simulink model "torqueBalancing2015a"  (Simulink 8.5)
settings: Solver=FixedStepDiscrete  StartTime=0.0  StopTime="CONFIG.SIMULATION_TIME "  FixedStep=CONFIG.Ts  RelTol=1e-3
InitFcn:
  | cd(fileparts(which(bdroot)));
  | initTorqueBalancing;
values from neighbouring files (symbols this model uses):
  WBT_modelName = 'matlabTorqueBalancing'    [initTorqueBalancing.m]
undefined symbols (not defined in the file or in its folder): bVectorConstraintsFeet, bVectorConstraintsLegs, CONFIG, ConstraintsMatrixFeet, ConstraintsMatrixLegs, DiscIntNeverNeededParam, gain, references, reg, ROBOT_DOF, ROBOT_DOF_FOR_SIMULINK, sat, SM, sm, WBT_robotName
libraries: WBToolboxLibrary x179, simulink x13
(part 3 of 4)

== system torqueBalancing2015a/DesValues/State Machine StandUp/w_H_root_link2 ==
  qj : Inport
  inertial : Inport  Port=2
  "CoM6D ->  CoMXYZ1" : Selector  NumberOfDimensions=2  InputPortWidth=7  IndexOptions=Index vector (dialog),Index vector (dialog)  Indices=[1 2 3],[1 2 3]  OutputSizes=1,1
  Constant2 : Constant  Value=eye(4)
  Constant5 : Constant  Value=eye(4)
  Constant6 : Constant  Value=eye(4)
  Inv\* : Product  Inputs=/*  Multiplication=Matrix(*)
  Inv\*1 : Product  Inputs=/*  Multiplication=Matrix(*)
  Inv\*2 : Product  Inputs=/  Multiplication=Matrix(*)
  Product : Product  Multiplication=Matrix(*)
  Selector : Selector  InputPortWidth=12  IndexOptions=Index vector (dialog)  Indices=[4 5 6 ]  OutputSizes=1
  Subsystem : Subsystem
  Switch6 : Switch  Criteria=u2 > Threshold
  USE_IMU4EST_BASE : Constant  Value=CONFIG.USE_IMU4EST_BASE
  fromImuToHomogeousTransformFCN : MATLAB Function  TreatAsAtomicUnit=on
      settings: PermitHierarchicalResolution=ParametersOnly
  holder 1 : WBToolboxLibrary/Utilities/holder 
  holder 2 : WBToolboxLibrary/Utilities/holder 
  imu : WBToolboxLibrary/wholeBodyModel/Kinematics/Forward Kinematics  frameName='imu_frame'  robotName=WBT_robotName  localName=WBT_modelName  wbiFile=WBT_wbiFilename  wbiList=WBT_wbiList
  l_sole_acc : Scope
      settings: TimeRange=60  ShowLegends=on  MaxDataPoints=5000  SaveToWorkspace=off  YMin=-4.47309  YMax=14.2668  SampleTime=-1
  link : WBToolboxLibrary/wholeBodyModel/Kinematics/Forward Kinematics  frameName=link_name  robotName=WBT_robotName  localName=WBT_modelName  wbiFile=WBT_wbiFilename  wbiList=WBT_wbiList
  root_link : WBToolboxLibrary/wholeBodyModel/Kinematics/Forward Kinematics  frameName='root_link'  robotName=WBT_robotName  localName=WBT_modelName  wbiFile=WBT_wbiFilename  wbiList=WBT_wbiList
  w_H_root : Outport
  wires:
  Constant5/1 -> imu/1
  Inv\*/1 -> holder 1/1, fromImuToHomogeousTransformFCN/1(imu_H_link), Inv\*2/1  "imu_H_link"
  imu/1 -> Inv\*/1
  Constant6/1 -> link/1
  Inv\*1/1 -> Switch6/3, fromImuToHomogeousTransformFCN/3(link_H_root)  "link_H_root"
  link/1 -> Inv\*1/1, Inv\*/2
  inertial/1 -> Selector/1, holder 2/1, fromImuToHomogeousTransformFCN/5(inertial)
  Switch6/1 -> w_H_root/1
  USE_IMU4EST_BASE/1 -> Switch6/2
  fromImuToHomogeousTransformFCN/1(w_H_root) -> Switch6/1
  Constant2/1 -> root_link/1
  qj/1 -> root_link/2, link/2, imu/2
  root_link/1 -> Inv\*1/2
  holder 1/1 -> fromImuToHomogeousTransformFCN/2(imu_H_link_0)
  holder 2/1 -> fromImuToHomogeousTransformFCN/4(inertial_0)
  Inv\*2/1 -> "CoM6D ->  CoMXYZ1"/1
  "CoM6D ->  CoMXYZ1"/1 -> Product/1  "l_sole_R_imu"
  Selector/1 -> Product/2  "imu_acce"
  Product/1 -> l_sole_acc/1
  Subsystem/1(Neck Position) -> fromImuToHomogeousTransformFCN/6(neck)

== system torqueBalancing2015a/DesValues/State Machine StandUp/xCom2 ==
  qj : Inport
  w_H_b : Inport  Port=2
  "CoM6D ->  CoMXYZ2" : Selector  NumberOfDimensions=2  InputPortWidth=7  IndexOptions=Index vector (dialog),Index vector (dialog)  Indices=[1 2 3],[4]  OutputSizes=1,1
  com : WBToolboxLibrary/wholeBodyModel/Kinematics/Forward Kinematics  frameName='com'  robotName=WBT_robotName  localName=WBT_modelName  wbiFile=WBT_wbiFilename  wbiList=WBT_wbiList
  xCom : Outport
  wires:
  qj/1 -> com/2
  "CoM6D ->  CoMXYZ2"/1 -> xCom/1
  com/1 -> "CoM6D ->  CoMXYZ2"/1
  w_H_b/1 -> com/1

== system torqueBalancing2015a/DesValues/State Machine Walking/Visualise extrnal wrenches   ==
  wL_WBDT : Inport
  wR_WBDT : Inport  Port=2
  Enable : EnablePort
  left foot ext wrench : Scope
      settings: TimeRange=auto  LimitDataPoints=on  MaxDataPoints=5000  SaveToWorkspace=off  YMin=-10  YMax=10  SampleTime=-1  DataFormat=Array
  right foot ext wrench : Scope
      settings: TimeRange=42.68  ShowLegends=on  MaxDataPoints=5000  SaveToWorkspace=off  SaveName=ScopeData2  YMin=-499.56546  YMax=285.33819  SampleTime=-1  DataFormat=Array
  wires:
  wR_WBDT/1 -> right foot ext wrench/1  "wR_WBDT"
  wL_WBDT/1 -> left foot ext wrench/1  "wL_WBDT"

== system torqueBalancing2015a/DesValues/State Machine Walking/nu ==
  qj : Inport
  w_H_b : Inport  Port=2
  "constraints " : Inport  Port=3
  Get Estimate : WBToolboxLibrary/wholeBodyStates/Get Estimate  estimateType=Joints Velocity  robotName=WBT_robotName  localName=WBT_modelName  wbiFile=WBT_wbiFilename  wbiList=WBT_wbiList
  Jacobian l_sole : WBToolboxLibrary/wholeBodyModel/Jacobians/Jacobian  frameName='l_sole'  robotName=WBT_robotName  localName=WBT_modelName  wbiFile=WBT_wbiFilename  wbiList=WBT_wbiList
  Jacobian r_sole : WBToolboxLibrary/wholeBodyModel/Jacobians/Jacobian  frameName='r_sole'  robotName=WBT_robotName  localName=WBT_modelName  wbiFile=WBT_wbiFilename  wbiList=WBT_wbiList
  MATLAB Function : MATLAB Function  TreatAsAtomicUnit=on
      settings: PermitHierarchicalResolution=ParametersOnly
  Mux : Mux  Inputs=2
  vb + Dqj : Outport
  wires:
  Get Estimate/1 -> MATLAB Function/4(qD), Mux/2
  Mux/1 -> vb + Dqj/1
  Jacobian r_sole/1 -> MATLAB Function/2(JcRightFoot)
  "constraints "/1 -> MATLAB Function/3(activeFeetConstraints)
  MATLAB Function/1(y) -> Mux/1
  Jacobian l_sole/1 -> MATLAB Function/1(JcLeftFoot)
  qj/1 -> Jacobian l_sole/2, Jacobian r_sole/2
  w_H_b/1 -> Jacobian r_sole/1, Jacobian l_sole/1

== system torqueBalancing2015a/DesValues/State Machine Walking/w_H_root_link1 ==
  qj : Inport
  inertial : Inport  Port=2
  "CoM6D ->  CoMXYZ1" : Selector  NumberOfDimensions=2  InputPortWidth=7  IndexOptions=Index vector (dialog),Index vector (dialog)  Indices=[1 2 3],[1 2 3]  OutputSizes=1,1
  Constant2 : Constant  Value=eye(4)
  Constant5 : Constant  Value=eye(4)
  Constant6 : Constant  Value=eye(4)
  Inv\* : Product  Inputs=/*  Multiplication=Matrix(*)
  Inv\*1 : Product  Inputs=/*  Multiplication=Matrix(*)
  Inv\*2 : Product  Inputs=/  Multiplication=Matrix(*)
  Product : Product  Multiplication=Matrix(*)
  Selector : Selector  InputPortWidth=12  IndexOptions=Index vector (dialog)  Indices=[4 5 6 ]  OutputSizes=1
  Subsystem : Subsystem
  Switch6 : Switch  Criteria=u2 > Threshold
  USE_IMU4EST_BASE : Constant  Value=CONFIG.USE_IMU4EST_BASE
  fromImuToHomogeousTransformFCN : MATLAB Function  TreatAsAtomicUnit=on
      settings: PermitHierarchicalResolution=ParametersOnly
  holder 1 : WBToolboxLibrary/Utilities/holder 
  holder 2 : WBToolboxLibrary/Utilities/holder 
  imu : WBToolboxLibrary/wholeBodyModel/Kinematics/Forward Kinematics  frameName='imu_frame'  robotName=WBT_robotName  localName=WBT_modelName  wbiFile=WBT_wbiFilename  wbiList=WBT_wbiList
  l_sole_acc : Scope
      settings: TimeRange=60  ShowLegends=on  MaxDataPoints=5000  SaveToWorkspace=off  YMin=-4.47309  YMax=14.2668  SampleTime=-1
  link : WBToolboxLibrary/wholeBodyModel/Kinematics/Forward Kinematics  frameName=link_name  robotName=WBT_robotName  localName=WBT_modelName  wbiFile=WBT_wbiFilename  wbiList=WBT_wbiList
  root_link : WBToolboxLibrary/wholeBodyModel/Kinematics/Forward Kinematics  frameName='root_link'  robotName=WBT_robotName  localName=WBT_modelName  wbiFile=WBT_wbiFilename  wbiList=WBT_wbiList
  w_H_root : Outport
  wires:
  Constant5/1 -> imu/1
  Inv\*/1 -> holder 1/1, fromImuToHomogeousTransformFCN/1(imu_H_link), Inv\*2/1  "imu_H_link"
  imu/1 -> Inv\*/1
  Constant6/1 -> link/1
  Inv\*1/1 -> Switch6/3, fromImuToHomogeousTransformFCN/3(link_H_root)  "link_H_root"
  link/1 -> Inv\*1/1, Inv\*/2
  inertial/1 -> Selector/1, holder 2/1, fromImuToHomogeousTransformFCN/5(inertial)
  Switch6/1 -> w_H_root/1
  USE_IMU4EST_BASE/1 -> Switch6/2
  fromImuToHomogeousTransformFCN/1(w_H_root) -> Switch6/1
  Constant2/1 -> root_link/1
  qj/1 -> root_link/2, link/2, imu/2
  root_link/1 -> Inv\*1/2
  holder 1/1 -> fromImuToHomogeousTransformFCN/2(imu_H_link_0)
  holder 2/1 -> fromImuToHomogeousTransformFCN/4(inertial_0)
  Inv\*2/1 -> "CoM6D ->  CoMXYZ1"/1
  "CoM6D ->  CoMXYZ1"/1 -> Product/1  "l_sole_R_imu"
  Selector/1 -> Product/2  "imu_acce"
  Product/1 -> l_sole_acc/1
  Subsystem/1(Neck Position) -> fromImuToHomogeousTransformFCN/6(neck)

== system torqueBalancing2015a/DesValues/State Machine Walking/w_H_root_link2 ==
  qj : Inport
  inertial : Inport  Port=2
  "CoM6D ->  CoMXYZ1" : Selector  NumberOfDimensions=2  InputPortWidth=7  IndexOptions=Index vector (dialog),Index vector (dialog)  Indices=[1 2 3],[1 2 3]  OutputSizes=1,1
  Constant2 : Constant  Value=eye(4)
  Constant5 : Constant  Value=eye(4)
  Constant6 : Constant  Value=eye(4)
  Inv\* : Product  Inputs=/*  Multiplication=Matrix(*)
  Inv\*1 : Product  Inputs=/*  Multiplication=Matrix(*)
  Inv\*2 : Product  Inputs=/  Multiplication=Matrix(*)
  Product : Product  Multiplication=Matrix(*)
  Selector : Selector  InputPortWidth=12  IndexOptions=Index vector (dialog)  Indices=[4 5 6 ]  OutputSizes=1
  Subsystem : Subsystem
  Switch6 : Switch  Criteria=u2 > Threshold
  USE_IMU4EST_BASE : Constant  Value=CONFIG.USE_IMU4EST_BASE
  fromImuToHomogeousTransformFCN : MATLAB Function  TreatAsAtomicUnit=on
      settings: PermitHierarchicalResolution=ParametersOnly
  holder 1 : WBToolboxLibrary/Utilities/holder 
  holder 2 : WBToolboxLibrary/Utilities/holder 
  imu : WBToolboxLibrary/wholeBodyModel/Kinematics/Forward Kinematics  frameName='imu_frame'  robotName=WBT_robotName  localName=WBT_modelName  wbiFile=WBT_wbiFilename  wbiList=WBT_wbiList
  l_sole_acc : Scope
      settings: TimeRange=60  ShowLegends=on  MaxDataPoints=5000  SaveToWorkspace=off  YMin=-4.47309  YMax=14.2668  SampleTime=-1
  link : WBToolboxLibrary/wholeBodyModel/Kinematics/Forward Kinematics  frameName=link_name  robotName=WBT_robotName  localName=WBT_modelName  wbiFile=WBT_wbiFilename  wbiList=WBT_wbiList
  root_link : WBToolboxLibrary/wholeBodyModel/Kinematics/Forward Kinematics  frameName='root_link'  robotName=WBT_robotName  localName=WBT_modelName  wbiFile=WBT_wbiFilename  wbiList=WBT_wbiList
  w_H_root : Outport
  wires:
  Constant5/1 -> imu/1
  Inv\*/1 -> holder 1/1, fromImuToHomogeousTransformFCN/1(imu_H_link), Inv\*2/1  "imu_H_link"
  imu/1 -> Inv\*/1
  Constant6/1 -> link/1
  Inv\*1/1 -> Switch6/3, fromImuToHomogeousTransformFCN/3(link_H_root)  "link_H_root"
  link/1 -> Inv\*1/1, Inv\*/2
  inertial/1 -> Selector/1, holder 2/1, fromImuToHomogeousTransformFCN/5(inertial)
  Switch6/1 -> w_H_root/1
  USE_IMU4EST_BASE/1 -> Switch6/2
  fromImuToHomogeousTransformFCN/1(w_H_root) -> Switch6/1
  Constant2/1 -> root_link/1
  qj/1 -> root_link/2, link/2, imu/2
  root_link/1 -> Inv\*1/2
  holder 1/1 -> fromImuToHomogeousTransformFCN/2(imu_H_link_0)
  holder 2/1 -> fromImuToHomogeousTransformFCN/4(inertial_0)
  Inv\*2/1 -> "CoM6D ->  CoMXYZ1"/1
  "CoM6D ->  CoMXYZ1"/1 -> Product/1  "l_sole_R_imu"
  Selector/1 -> Product/2  "imu_acce"
  Product/1 -> l_sole_acc/1
  Subsystem/1(Neck Position) -> fromImuToHomogeousTransformFCN/6(neck)

== system torqueBalancing2015a/DesValues/State Machine Walking/xCom ==
  qj : Inport
  w_H_b : Inport  Port=2
  "CoM6D ->  CoMXYZ2" : Selector  NumberOfDimensions=2  InputPortWidth=7  IndexOptions=Index vector (dialog),Index vector (dialog)  Indices=[1 2 3],[4]  OutputSizes=1,1
  com : WBToolboxLibrary/wholeBodyModel/Kinematics/Forward Kinematics  frameName='com'  robotName=WBT_robotName  localName=WBT_modelName  wbiFile=WBT_wbiFilename  wbiList=WBT_wbiList
  xCom : Outport
  wires:
  qj/1 -> com/2
  "CoM6D ->  CoMXYZ2"/1 -> xCom/1
  com/1 -> "CoM6D ->  CoMXYZ2"/1
  w_H_b/1 -> com/1

== system torqueBalancing2015a/DesValues/State Machine Walking/xCom1 ==
  qj : Inport
  w_H_b : Inport  Port=2
  "CoM6D ->  CoMXYZ2" : Selector  NumberOfDimensions=2  InputPortWidth=7  IndexOptions=Index vector (dialog),Index vector (dialog)  Indices=[1 2 3],[4]  OutputSizes=1,1
  com : WBToolboxLibrary/wholeBodyModel/Kinematics/Forward Kinematics  frameName='com'  robotName=WBT_robotName  localName=WBT_modelName  wbiFile=WBT_wbiFilename  wbiList=WBT_wbiList
  xCom : Outport
  wires:
  qj/1 -> com/2
  "CoM6D ->  CoMXYZ2"/1 -> xCom/1
  com/1 -> "CoM6D ->  CoMXYZ2"/1
  w_H_b/1 -> com/1

== system torqueBalancing2015a/controller_QP/QP/Visualize eventual QP failures ==
  exitFlagQP : Inport
  state : Inport  Port=2
  Enable : EnablePort
  "QP status (0: no failure, 1: not using)" : Scope  NumInputPorts=2
      settings: TimeRange=auto  ShowLegends=on  MaxDataPoints=5000  SaveName=QPStatus  YMin=-2.25~0.625  YMax=0.25~4.375  SampleTime=-1
  wires:
  exitFlagQP/1 -> "QP status (0: no failure, 1: not using)"/1  "exitFlagQP"
  state/1 -> "QP status (0: no failure, 1: not using)"/2

== system torqueBalancing2015a/controller_QP/integralOf Hw1/w_H_root_link1 ==
  qj : Inport
  inertial : Inport  Port=2
  "CoM6D ->  CoMXYZ1" : Selector  NumberOfDimensions=2  InputPortWidth=7  IndexOptions=Index vector (dialog),Index vector (dialog)  Indices=[1 2 3],[1 2 3]  OutputSizes=1,1
  Constant2 : Constant  Value=eye(4)
  Constant5 : Constant  Value=eye(4)
  Constant6 : Constant  Value=eye(4)
  Inv\* : Product  Inputs=/*  Multiplication=Matrix(*)
  Inv\*1 : Product  Inputs=/*  Multiplication=Matrix(*)
  Inv\*2 : Product  Inputs=/  Multiplication=Matrix(*)
  Product : Product  Multiplication=Matrix(*)
  Selector : Selector  InputPortWidth=12  IndexOptions=Index vector (dialog)  Indices=[4 5 6 ]  OutputSizes=1
  Subsystem : Subsystem
  Switch6 : Switch  Criteria=u2 > Threshold
  USE_IMU4EST_BASE : Constant  Value=CONFIG.USE_IMU4EST_BASE
  fromImuToHomogeousTransformFCN : MATLAB Function  TreatAsAtomicUnit=on
      settings: PermitHierarchicalResolution=ParametersOnly
  holder 1 : WBToolboxLibrary/Utilities/holder 
  holder 2 : WBToolboxLibrary/Utilities/holder 
  imu : WBToolboxLibrary/wholeBodyModel/Kinematics/Forward Kinematics  frameName='imu_frame'  robotName=WBT_robotName  localName=WBT_modelName  wbiFile=WBT_wbiFilename  wbiList=WBT_wbiList
  l_sole_acc : Scope
      settings: TimeRange=60  ShowLegends=on  MaxDataPoints=5000  SaveToWorkspace=off  YMin=-4.47309  YMax=14.2668  SampleTime=-1
  link : WBToolboxLibrary/wholeBodyModel/Kinematics/Forward Kinematics  frameName=link_name  robotName=WBT_robotName  localName=WBT_modelName  wbiFile=WBT_wbiFilename  wbiList=WBT_wbiList
  root_link : WBToolboxLibrary/wholeBodyModel/Kinematics/Forward Kinematics  frameName='root_link'  robotName=WBT_robotName  localName=WBT_modelName  wbiFile=WBT_wbiFilename  wbiList=WBT_wbiList
  w_H_root : Outport
  wires:
  Constant5/1 -> imu/1
  Inv\*/1 -> holder 1/1, fromImuToHomogeousTransformFCN/1(imu_H_link), Inv\*2/1  "imu_H_link"
  imu/1 -> Inv\*/1
  Constant6/1 -> link/1
  Inv\*1/1 -> Switch6/3, fromImuToHomogeousTransformFCN/3(link_H_root)  "link_H_root"
  link/1 -> Inv\*1/1, Inv\*/2
  inertial/1 -> Selector/1, holder 2/1, fromImuToHomogeousTransformFCN/5(inertial)
  Switch6/1 -> w_H_root/1
  USE_IMU4EST_BASE/1 -> Switch6/2
  fromImuToHomogeousTransformFCN/1(w_H_root) -> Switch6/1
  Constant2/1 -> root_link/1
  qj/1 -> root_link/2, link/2, imu/2
  root_link/1 -> Inv\*1/2
  holder 1/1 -> fromImuToHomogeousTransformFCN/2(imu_H_link_0)
  holder 2/1 -> fromImuToHomogeousTransformFCN/4(inertial_0)
  Inv\*2/1 -> "CoM6D ->  CoMXYZ1"/1
  "CoM6D ->  CoMXYZ1"/1 -> Product/1  "l_sole_R_imu"
  Selector/1 -> Product/2  "imu_acce"
  Product/1 -> l_sole_acc/1
  Subsystem/1(Neck Position) -> fromImuToHomogeousTransformFCN/6(neck)

== system torqueBalancing2015a/controller_QP/integralOf Hw1/w_H_root_link2 ==
  qj : Inport
  inertial : Inport  Port=2
  "CoM6D ->  CoMXYZ1" : Selector  NumberOfDimensions=2  InputPortWidth=7  IndexOptions=Index vector (dialog),Index vector (dialog)  Indices=[1 2 3],[1 2 3]  OutputSizes=1,1
  Constant2 : Constant  Value=eye(4)
  Constant5 : Constant  Value=eye(4)
  Constant6 : Constant  Value=eye(4)
  Inv\* : Product  Inputs=/*  Multiplication=Matrix(*)
  Inv\*1 : Product  Inputs=/*  Multiplication=Matrix(*)
  Inv\*2 : Product  Inputs=/  Multiplication=Matrix(*)
  Product : Product  Multiplication=Matrix(*)
  Selector : Selector  InputPortWidth=12  IndexOptions=Index vector (dialog)  Indices=[4 5 6 ]  OutputSizes=1
  Subsystem : Subsystem
  Switch6 : Switch  Criteria=u2 > Threshold
  USE_IMU4EST_BASE : Constant  Value=CONFIG.USE_IMU4EST_BASE
  fromImuToHomogeousTransformFCN : MATLAB Function  TreatAsAtomicUnit=on
      settings: PermitHierarchicalResolution=ParametersOnly
  holder 1 : WBToolboxLibrary/Utilities/holder 
  holder 2 : WBToolboxLibrary/Utilities/holder 
  imu : WBToolboxLibrary/wholeBodyModel/Kinematics/Forward Kinematics  frameName='imu_frame'  robotName=WBT_robotName  localName=WBT_modelName  wbiFile=WBT_wbiFilename  wbiList=WBT_wbiList
  l_sole_acc : Scope
      settings: TimeRange=60  ShowLegends=on  MaxDataPoints=5000  SaveToWorkspace=off  YMin=-4.47309  YMax=14.2668  SampleTime=-1
  link : WBToolboxLibrary/wholeBodyModel/Kinematics/Forward Kinematics  frameName=link_name  robotName=WBT_robotName  localName=WBT_modelName  wbiFile=WBT_wbiFilename  wbiList=WBT_wbiList
  root_link : WBToolboxLibrary/wholeBodyModel/Kinematics/Forward Kinematics  frameName='root_link'  robotName=WBT_robotName  localName=WBT_modelName  wbiFile=WBT_wbiFilename  wbiList=WBT_wbiList
  w_H_root : Outport
  wires:
  Constant5/1 -> imu/1
  Inv\*/1 -> holder 1/1, fromImuToHomogeousTransformFCN/1(imu_H_link), Inv\*2/1  "imu_H_link"
  imu/1 -> Inv\*/1
  Constant6/1 -> link/1
  Inv\*1/1 -> Switch6/3, fromImuToHomogeousTransformFCN/3(link_H_root)  "link_H_root"
  link/1 -> Inv\*1/1, Inv\*/2
  inertial/1 -> Selector/1, holder 2/1, fromImuToHomogeousTransformFCN/5(inertial)
  Switch6/1 -> w_H_root/1
  USE_IMU4EST_BASE/1 -> Switch6/2
  fromImuToHomogeousTransformFCN/1(w_H_root) -> Switch6/1
  Constant2/1 -> root_link/1
  qj/1 -> root_link/2, link/2, imu/2
  root_link/1 -> Inv\*1/2
  holder 1/1 -> fromImuToHomogeousTransformFCN/2(imu_H_link_0)
  holder 2/1 -> fromImuToHomogeousTransformFCN/4(inertial_0)
  Inv\*2/1 -> "CoM6D ->  CoMXYZ1"/1
  "CoM6D ->  CoMXYZ1"/1 -> Product/1  "l_sole_R_imu"
  Selector/1 -> Product/2  "imu_acce"
  Product/1 -> l_sole_acc/1
  Subsystem/1(Neck Position) -> fromImuToHomogeousTransformFCN/6(neck)

== system torqueBalancing2015a/DesValues/Internal coordinator/w_H_root_link1/Subsystem ==
  Constant : Constant  Value=zeros(3,1)
  Gain : Gain  Gain=pi/180
  Head state : WBToolboxLibrary/Utilities/Yarp Read  portName=['/',WBT_robotName, '/head/state:o']  signalSize=6  blocking=off  timestamp=off  autoconnect=on  errorOnConnection=off
  Selector1 : Selector  InputPortWidth=6  IndexOptions=Index vector (dialog)  Indices=[1:3]  OutputSizes=1
  Switch : Switch  Criteria=u2 > Threshold
  USE_IMU4EST_BASE1 : Constant  Value=CONFIG.CORRECT_NECK_IMU
  Neck Position : Outport
  wires:
  Head state/1 -> Gain/1
  Selector1/1 -> Switch/1  "neck"
  USE_IMU4EST_BASE1/1 -> Switch/2
  Switch/1 -> Neck Position/1
  Gain/1 -> Selector1/1
  Constant/1 -> Switch/3

== system torqueBalancing2015a/DesValues/State Machine/visualise inertial/Visualize hom transf2 ==
  H : Inport
  "CoM6D ->  CoMXYZ1" : Selector  NumberOfDimensions=2  InputPortWidth=7  IndexOptions=Index vector (dialog),Index vector (dialog)  Indices=[1 2 3],[1 2 3]  OutputSizes=1,1
  "CoM6D ->  CoMXYZ2" : Selector  NumberOfDimensions=2  InputPortWidth=7  IndexOptions=Index vector (dialog),Index vector (dialog)  Indices=[1 2 3],[4]  OutputSizes=1,1
  Hom : Scope
      settings: TimeRange=auto  ShowLegends=on  MaxDataPoints=5000  SaveToWorkspace=off  SaveName=ScopeData3  YMin=-0.02533  YMax=0.01393  SampleTime=-1
  MATLAB Function : MATLAB Function  TreatAsAtomicUnit=on
      settings: PermitHierarchicalResolution=ParametersOnly
  p : Scope
      settings: TimeRange=auto  MaxDataPoints=5000  SaveToWorkspace=off  SaveName=ScopeData2  YMin=-0.05005  YMax=0.09732  SampleTime=-1
  rollPitchYaw : Scope
      settings: TimeRange=auto  ShowLegends=on  MaxDataPoints=5000  SaveToWorkspace=off  YMin=-0.15453  YMax=0.04472  SampleTime=-1
  wires:
  "CoM6D ->  CoMXYZ2"/1 -> p/1
  H/1 -> "CoM6D ->  CoMXYZ2"/1, Hom/1, "CoM6D ->  CoMXYZ1"/1
  "CoM6D ->  CoMXYZ1"/1 -> MATLAB Function/1(R)
  MATLAB Function/1(rollPitchYaw) -> rollPitchYaw/1

== system torqueBalancing2015a/DesValues/State Machine/visualise inertial/Visualize hom transf4 ==
  H : Inport
  "CoM6D ->  CoMXYZ1" : Selector  NumberOfDimensions=2  InputPortWidth=7  IndexOptions=Index vector (dialog),Index vector (dialog)  Indices=[1 2 3],[1 2 3]  OutputSizes=1,1
  "CoM6D ->  CoMXYZ2" : Selector  NumberOfDimensions=2  InputPortWidth=7  IndexOptions=Index vector (dialog),Index vector (dialog)  Indices=[1 2 3],[4]  OutputSizes=1,1
  Hom : Scope
      settings: TimeRange=auto  ShowLegends=on  MaxDataPoints=5000  SaveToWorkspace=off  SaveName=ScopeData3  YMin=-0.02533  YMax=0.01393  SampleTime=-1
  MATLAB Function : MATLAB Function  TreatAsAtomicUnit=on
      settings: PermitHierarchicalResolution=ParametersOnly
  p : Scope
      settings: TimeRange=auto  MaxDataPoints=5000  SaveToWorkspace=off  SaveName=ScopeData2  YMin=-0.05005  YMax=0.09732  SampleTime=-1
  rollPitchYaw : Scope
      settings: TimeRange=auto  ShowLegends=on  MaxDataPoints=5000  SaveToWorkspace=off  YMin=-0.15453  YMax=0.04472  SampleTime=-1
  wires:
  "CoM6D ->  CoMXYZ2"/1 -> p/1
  H/1 -> "CoM6D ->  CoMXYZ2"/1, Hom/1, "CoM6D ->  CoMXYZ1"/1
  "CoM6D ->  CoMXYZ1"/1 -> MATLAB Function/1(R)
  MATLAB Function/1(rollPitchYaw) -> rollPitchYaw/1

== system torqueBalancing2015a/DesValues/State Machine/visualise inertial/Visualize hom transf5 ==
  H : Inport
  "CoM6D ->  CoMXYZ1" : Selector  NumberOfDimensions=2  InputPortWidth=7  IndexOptions=Index vector (dialog),Index vector (dialog)  Indices=[1 2 3],[1 2 3]  OutputSizes=1,1
  "CoM6D ->  CoMXYZ2" : Selector  NumberOfDimensions=2  InputPortWidth=7  IndexOptions=Index vector (dialog),Index vector (dialog)  Indices=[1 2 3],[4]  OutputSizes=1,1
  Hom : Scope
      settings: TimeRange=auto  ShowLegends=on  MaxDataPoints=5000  SaveToWorkspace=off  SaveName=ScopeData3  YMin=-0.02533  YMax=0.01393  SampleTime=-1
  MATLAB Function : MATLAB Function  TreatAsAtomicUnit=on
      settings: PermitHierarchicalResolution=ParametersOnly
  p : Scope
      settings: TimeRange=auto  MaxDataPoints=5000  SaveToWorkspace=off  SaveName=ScopeData2  YMin=-0.05005  YMax=0.09732  SampleTime=-1
  rollPitchYaw : Scope
      settings: TimeRange=auto  ShowLegends=on  MaxDataPoints=5000  SaveToWorkspace=off  YMin=-0.15453  YMax=0.04472  SampleTime=-1
  wires:
  "CoM6D ->  CoMXYZ2"/1 -> p/1
  H/1 -> "CoM6D ->  CoMXYZ2"/1, Hom/1, "CoM6D ->  CoMXYZ1"/1
  "CoM6D ->  CoMXYZ1"/1 -> MATLAB Function/1(R)
  MATLAB Function/1(rollPitchYaw) -> rollPitchYaw/1

== system torqueBalancing2015a/DesValues/State Machine/visualise inertial/Visualize hom transf6 ==
  H : Inport
  "CoM6D ->  CoMXYZ1" : Selector  NumberOfDimensions=2  InputPortWidth=7  IndexOptions=Index vector (dialog),Index vector (dialog)  Indices=[1 2 3],[1 2 3]  OutputSizes=1,1
  "CoM6D ->  CoMXYZ2" : Selector  NumberOfDimensions=2  InputPortWidth=7  IndexOptions=Index vector (dialog),Index vector (dialog)  Indices=[1 2 3],[4]  OutputSizes=1,1
  Hom : Scope
      settings: TimeRange=auto  ShowLegends=on  MaxDataPoints=5000  SaveToWorkspace=off  SaveName=ScopeData3  YMin=-0.02533  YMax=0.01393  SampleTime=-1
  MATLAB Function : MATLAB Function  TreatAsAtomicUnit=on
      settings: PermitHierarchicalResolution=ParametersOnly
  p : Scope
      settings: TimeRange=auto  MaxDataPoints=5000  SaveToWorkspace=off  SaveName=ScopeData2  YMin=-0.05005  YMax=0.09732  SampleTime=-1
  rollPitchYaw : Scope
      settings: TimeRange=auto  ShowLegends=on  MaxDataPoints=5000  SaveToWorkspace=off  YMin=-0.15453  YMax=0.04472  SampleTime=-1
  wires:
  "CoM6D ->  CoMXYZ2"/1 -> p/1
  H/1 -> "CoM6D ->  CoMXYZ2"/1, Hom/1, "CoM6D ->  CoMXYZ1"/1
  "CoM6D ->  CoMXYZ1"/1 -> MATLAB Function/1(R)
  MATLAB Function/1(rollPitchYaw) -> rollPitchYaw/1

== system torqueBalancing2015a/DesValues/State Machine/visualise inertial/Visualize hom transf7 ==
  H : Inport
  "CoM6D ->  CoMXYZ1" : Selector  NumberOfDimensions=2  InputPortWidth=7  IndexOptions=Index vector (dialog),Index vector (dialog)  Indices=[1 2 3],[1 2 3]  OutputSizes=1,1
  "CoM6D ->  CoMXYZ2" : Selector  NumberOfDimensions=2  InputPortWidth=7  IndexOptions=Index vector (dialog),Index vector (dialog)  Indices=[1 2 3],[4]  OutputSizes=1,1
  Hom : Scope
      settings: TimeRange=auto  ShowLegends=on  MaxDataPoints=5000  SaveToWorkspace=off  SaveName=ScopeData3  YMin=-0.02533  YMax=0.01393  SampleTime=-1
  MATLAB Function : MATLAB Function  TreatAsAtomicUnit=on
      settings: PermitHierarchicalResolution=ParametersOnly
  p : Scope
      settings: TimeRange=auto  MaxDataPoints=5000  SaveToWorkspace=off  SaveName=ScopeData2  YMin=-0.05005  YMax=0.09732  SampleTime=-1
  rollPitchYaw : Scope
      settings: TimeRange=auto  ShowLegends=on  MaxDataPoints=5000  SaveToWorkspace=off  YMin=-0.15453  YMax=0.04472  SampleTime=-1
  wires:
  "CoM6D ->  CoMXYZ2"/1 -> p/1
  H/1 -> "CoM6D ->  CoMXYZ2"/1, Hom/1, "CoM6D ->  CoMXYZ1"/1
  "CoM6D ->  CoMXYZ1"/1 -> MATLAB Function/1(R)
  MATLAB Function/1(rollPitchYaw) -> rollPitchYaw/1

== system torqueBalancing2015a/DesValues/State Machine/visualise inertial/Visualize hom transf8 ==
  H : Inport
  "CoM6D ->  CoMXYZ1" : Selector  NumberOfDimensions=2  InputPortWidth=7  IndexOptions=Index vector (dialog),Index vector (dialog)  Indices=[1 2 3],[1 2 3]  OutputSizes=1,1
  "CoM6D ->  CoMXYZ2" : Selector  NumberOfDimensions=2  InputPortWidth=7  IndexOptions=Index vector (dialog),Index vector (dialog)  Indices=[1 2 3],[4]  OutputSizes=1,1
  Hom : Scope
      settings: TimeRange=auto  ShowLegends=on  MaxDataPoints=5000  SaveToWorkspace=off  SaveName=ScopeData3  YMin=-0.02533  YMax=0.01393  SampleTime=-1
  MATLAB Function : MATLAB Function  TreatAsAtomicUnit=on
      settings: PermitHierarchicalResolution=ParametersOnly
  p : Scope
      settings: TimeRange=auto  MaxDataPoints=5000  SaveToWorkspace=off  SaveName=ScopeData2  YMin=-0.05005  YMax=0.09732  SampleTime=-1
  rollPitchYaw : Scope
      settings: TimeRange=auto  ShowLegends=on  MaxDataPoints=5000  SaveToWorkspace=off  YMin=-0.15453  YMax=0.04472  SampleTime=-1
  wires:
  "CoM6D ->  CoMXYZ2"/1 -> p/1
  H/1 -> "CoM6D ->  CoMXYZ2"/1, Hom/1, "CoM6D ->  CoMXYZ1"/1
  "CoM6D ->  CoMXYZ1"/1 -> MATLAB Function/1(R)
  MATLAB Function/1(rollPitchYaw) -> rollPitchYaw/1

== system torqueBalancing2015a/DesValues/State Machine/visualise inertial/l_sole_H_root_link2 ==
  qj : Inport
  Constant5 : Constant  Value=eye(4)
  Constant6 : Constant  Value=eye(4)
  Inv\* : Product  Inputs=/*  Multiplication=Matrix(*)
  Visualize hom transf4 : Subsystem
  link_name : WBToolboxLibrary/wholeBodyModel/Kinematics/Forward Kinematics  frameName=link_name  robotName=WBT_robotName  localName=WBT_modelName  wbiFile=WBT_wbiFilename  wbiList=WBT_wbiList
  root_link : WBToolboxLibrary/wholeBodyModel/Kinematics/Forward Kinematics  frameName='root_link'  robotName=WBT_robotName  localName=WBT_modelName  wbiFile=WBT_wbiFilename  wbiList=WBT_wbiList
  link_name_H_root_link : Outport
  wires:
  Constant5/1 -> link_name/1
  Inv\*/1 -> link_name_H_root_link/1  "link_name_H_root_link"
  link_name/1 -> Inv\*/1
  Constant6/1 -> root_link/1
  qj/1 -> link_name/2, root_link/2
  root_link/1 -> Visualize hom transf4/1(H), Inv\*/2

== system torqueBalancing2015a/DesValues/State Machine/visualise inertial/l_sole_H_root_link3 ==
  qj : Inport
  Constant5 : Constant  Value=eye(4)
  Constant6 : Constant  Value=eye(4)
  Inv\* : Product  Inputs=/*  Multiplication=Matrix(*)
  Visualize hom transf4 : Subsystem
  link_name : WBToolboxLibrary/wholeBodyModel/Kinematics/Forward Kinematics  frameName=link_name  robotName=WBT_robotName  localName=WBT_modelName  wbiFile=WBT_wbiFilename  wbiList=WBT_wbiList
  root_link : WBToolboxLibrary/wholeBodyModel/Kinematics/Forward Kinematics  frameName='root_link'  robotName=WBT_robotName  localName=WBT_modelName  wbiFile=WBT_wbiFilename  wbiList=WBT_wbiList
  link_name_H_root_link : Outport
  wires:
  Constant5/1 -> link_name/1
  Inv\*/1 -> link_name_H_root_link/1  "link_name_H_root_link"
  link_name/1 -> Inv\*/1
  Constant6/1 -> root_link/1
  qj/1 -> link_name/2, root_link/2
  root_link/1 -> Visualize hom transf4/1(H), Inv\*/2

== system torqueBalancing2015a/DesValues/State Machine/visualise inertial/w_H_root_link1 ==
  qj : Inport
  inertial : Inport  Port=2
  "CoM6D ->  CoMXYZ1" : Selector  NumberOfDimensions=2  InputPortWidth=7  IndexOptions=Index vector (dialog),Index vector (dialog)  Indices=[1 2 3],[1 2 3]  OutputSizes=1,1
  Constant2 : Constant  Value=eye(4)
  Constant5 : Constant  Value=eye(4)
  Constant6 : Constant  Value=eye(4)
  Inv\* : Product  Inputs=/*  Multiplication=Matrix(*)
  Inv\*1 : Product  Inputs=/*  Multiplication=Matrix(*)
  Inv\*2 : Product  Inputs=/  Multiplication=Matrix(*)
  Product : Product  Multiplication=Matrix(*)
  Selector : Selector  InputPortWidth=12  IndexOptions=Index vector (dialog)  Indices=[4 5 6 ]  OutputSizes=1
  Subsystem : Subsystem
  Switch6 : Switch  Criteria=u2 > Threshold
  USE_IMU4EST_BASE : Constant  Value=CONFIG.USE_IMU4EST_BASE
  fromImuToHomogeousTransformFCN : MATLAB Function  TreatAsAtomicUnit=on
      settings: PermitHierarchicalResolution=ParametersOnly
  holder 1 : WBToolboxLibrary/Utilities/holder 
  holder 2 : WBToolboxLibrary/Utilities/holder 
  imu : WBToolboxLibrary/wholeBodyModel/Kinematics/Forward Kinematics  frameName='imu_frame'  robotName=WBT_robotName  localName=WBT_modelName  wbiFile=WBT_wbiFilename  wbiList=WBT_wbiList
  l_sole_acc : Scope
      settings: TimeRange=60  ShowLegends=on  MaxDataPoints=5000  SaveToWorkspace=off  YMin=-4.47309  YMax=14.2668  SampleTime=-1
  link : WBToolboxLibrary/wholeBodyModel/Kinematics/Forward Kinematics  frameName=link_name  robotName=WBT_robotName  localName=WBT_modelName  wbiFile=WBT_wbiFilename  wbiList=WBT_wbiList
  root_link : WBToolboxLibrary/wholeBodyModel/Kinematics/Forward Kinematics  frameName='root_link'  robotName=WBT_robotName  localName=WBT_modelName  wbiFile=WBT_wbiFilename  wbiList=WBT_wbiList
  w_H_root : Outport
  wires:
  Constant5/1 -> imu/1
  Inv\*/1 -> holder 1/1, fromImuToHomogeousTransformFCN/1(imu_H_link), Inv\*2/1  "imu_H_link"
  imu/1 -> Inv\*/1
  Constant6/1 -> link/1
  Inv\*1/1 -> Switch6/3, fromImuToHomogeousTransformFCN/3(link_H_root)  "link_H_root"
  link/1 -> Inv\*1/1, Inv\*/2
  inertial/1 -> Selector/1, holder 2/1, fromImuToHomogeousTransformFCN/5(inertial)
  Switch6/1 -> w_H_root/1
  USE_IMU4EST_BASE/1 -> Switch6/2
  fromImuToHomogeousTransformFCN/1(w_H_root) -> Switch6/1
  Constant2/1 -> root_link/1
  qj/1 -> root_link/2, link/2, imu/2
  root_link/1 -> Inv\*1/2
  holder 1/1 -> fromImuToHomogeousTransformFCN/2(imu_H_link_0)
  holder 2/1 -> fromImuToHomogeousTransformFCN/4(inertial_0)
  Inv\*2/1 -> "CoM6D ->  CoMXYZ1"/1
  "CoM6D ->  CoMXYZ1"/1 -> Product/1  "l_sole_R_imu"
  Selector/1 -> Product/2  "imu_acce"
  Product/1 -> l_sole_acc/1
  Subsystem/1(Neck Position) -> fromImuToHomogeousTransformFCN/6(neck)

== system torqueBalancing2015a/DesValues/State Machine/visualise inertial/w_H_root_link3 ==
  qj : Inport
  inertial : Inport  Port=2
  "CoM6D ->  CoMXYZ1" : Selector  NumberOfDimensions=2  InputPortWidth=7  IndexOptions=Index vector (dialog),Index vector (dialog)  Indices=[1 2 3],[1 2 3]  OutputSizes=1,1
  Constant2 : Constant  Value=eye(4)
  Constant5 : Constant  Value=eye(4)
  Constant6 : Constant  Value=eye(4)
  Inv\* : Product  Inputs=/*  Multiplication=Matrix(*)
  Inv\*1 : Product  Inputs=/*  Multiplication=Matrix(*)
  Inv\*2 : Product  Inputs=/  Multiplication=Matrix(*)
  Product : Product  Multiplication=Matrix(*)
  Selector : Selector  InputPortWidth=12  IndexOptions=Index vector (dialog)  Indices=[4 5 6 ]  OutputSizes=1
  Subsystem : Subsystem
  Switch6 : Switch  Criteria=u2 > Threshold
  USE_IMU4EST_BASE : Constant  Value=CONFIG.USE_IMU4EST_BASE
  fromImuToHomogeousTransformFCN : MATLAB Function  TreatAsAtomicUnit=on
      settings: PermitHierarchicalResolution=ParametersOnly
  holder 1 : WBToolboxLibrary/Utilities/holder 
  holder 2 : WBToolboxLibrary/Utilities/holder 
  imu : WBToolboxLibrary/wholeBodyModel/Kinematics/Forward Kinematics  frameName='imu_frame'  robotName=WBT_robotName  localName=WBT_modelName  wbiFile=WBT_wbiFilename  wbiList=WBT_wbiList
  l_sole_acc : Scope
      settings: TimeRange=60  ShowLegends=on  MaxDataPoints=5000  SaveToWorkspace=off  YMin=-4.47309  YMax=14.2668  SampleTime=-1
  link : WBToolboxLibrary/wholeBodyModel/Kinematics/Forward Kinematics  frameName=link_name  robotName=WBT_robotName  localName=WBT_modelName  wbiFile=WBT_wbiFilename  wbiList=WBT_wbiList
  root_link : WBToolboxLibrary/wholeBodyModel/Kinematics/Forward Kinematics  frameName='root_link'  robotName=WBT_robotName  localName=WBT_modelName  wbiFile=WBT_wbiFilename  wbiList=WBT_wbiList
  w_H_root : Outport
  wires:
  Constant5/1 -> imu/1
  Inv\*/1 -> holder 1/1, fromImuToHomogeousTransformFCN/1(imu_H_link), Inv\*2/1  "imu_H_link"
  imu/1 -> Inv\*/1
  Constant6/1 -> link/1
  Inv\*1/1 -> Switch6/3, fromImuToHomogeousTransformFCN/3(link_H_root)  "link_H_root"
  link/1 -> Inv\*1/1, Inv\*/2
  inertial/1 -> Selector/1, holder 2/1, fromImuToHomogeousTransformFCN/5(inertial)
  Switch6/1 -> w_H_root/1
  USE_IMU4EST_BASE/1 -> Switch6/2
  fromImuToHomogeousTransformFCN/1(w_H_root) -> Switch6/1
  Constant2/1 -> root_link/1
  qj/1 -> root_link/2, link/2, imu/2
  root_link/1 -> Inv\*1/2
  holder 1/1 -> fromImuToHomogeousTransformFCN/2(imu_H_link_0)
  holder 2/1 -> fromImuToHomogeousTransformFCN/4(inertial_0)
  Inv\*2/1 -> "CoM6D ->  CoMXYZ1"/1
  "CoM6D ->  CoMXYZ1"/1 -> Product/1  "l_sole_R_imu"
  Selector/1 -> Product/2  "imu_acce"
  Product/1 -> l_sole_acc/1
  Subsystem/1(Neck Position) -> fromImuToHomogeousTransformFCN/6(neck)

== system torqueBalancing2015a/DesValues/State Machine/w_H_root_link1/Subsystem ==
  Constant : Constant  Value=zeros(3,1)
  Gain : Gain  Gain=pi/180
  Head state : WBToolboxLibrary/Utilities/Yarp Read  portName=['/',WBT_robotName, '/head/state:o']  signalSize=6  blocking=off  timestamp=off  autoconnect=on  errorOnConnection=off
  Selector1 : Selector  InputPortWidth=6  IndexOptions=Index vector (dialog)  Indices=[1:3]  OutputSizes=1
  Switch : Switch  Criteria=u2 > Threshold
  USE_IMU4EST_BASE1 : Constant  Value=CONFIG.CORRECT_NECK_IMU
  Neck Position : Outport
  wires:
  Head state/1 -> Gain/1
  Selector1/1 -> Switch/1  "neck"
  USE_IMU4EST_BASE1/1 -> Switch/2
  Switch/1 -> Neck Position/1
  Gain/1 -> Selector1/1
  Constant/1 -> Switch/3

== system torqueBalancing2015a/DesValues/State Machine/w_H_root_link2/Subsystem ==
  Constant : Constant  Value=zeros(3,1)
  Gain : Gain  Gain=pi/180
  Head state : WBToolboxLibrary/Utilities/Yarp Read  portName=['/',WBT_robotName, '/head/state:o']  signalSize=6  blocking=off  timestamp=off  autoconnect=on  errorOnConnection=off
  Selector1 : Selector  InputPortWidth=6  IndexOptions=Index vector (dialog)  Indices=[1:3]  OutputSizes=1
  Switch : Switch  Criteria=u2 > Threshold
  USE_IMU4EST_BASE1 : Constant  Value=CONFIG.CORRECT_NECK_IMU
  Neck Position : Outport
  wires:
  Head state/1 -> Gain/1
  Selector1/1 -> Switch/1  "neck"
  USE_IMU4EST_BASE1/1 -> Switch/2
  Switch/1 -> Neck Position/1
  Gain/1 -> Selector1/1
  Constant/1 -> Switch/3

== system torqueBalancing2015a/DesValues/State Machine StandUp/visualise inertial/Visualize hom transf2 ==
  H : Inport
  "CoM6D ->  CoMXYZ1" : Selector  NumberOfDimensions=2  InputPortWidth=7  IndexOptions=Index vector (dialog),Index vector (dialog)  Indices=[1 2 3],[1 2 3]  OutputSizes=1,1
  "CoM6D ->  CoMXYZ2" : Selector  NumberOfDimensions=2  InputPortWidth=7  IndexOptions=Index vector (dialog),Index vector (dialog)  Indices=[1 2 3],[4]  OutputSizes=1,1
  Hom : Scope
      settings: TimeRange=auto  ShowLegends=on  MaxDataPoints=5000  SaveToWorkspace=off  SaveName=ScopeData3  YMin=-0.02533  YMax=0.01393  SampleTime=-1
  MATLAB Function : MATLAB Function  TreatAsAtomicUnit=on
      settings: PermitHierarchicalResolution=ParametersOnly
  p : Scope
      settings: TimeRange=auto  MaxDataPoints=5000  SaveToWorkspace=off  SaveName=ScopeData2  YMin=-0.05005  YMax=0.09732  SampleTime=-1
  rollPitchYaw : Scope
      settings: TimeRange=auto  ShowLegends=on  MaxDataPoints=5000  SaveToWorkspace=off  YMin=-0.15453  YMax=0.04472  SampleTime=-1
  wires:
  "CoM6D ->  CoMXYZ2"/1 -> p/1
  H/1 -> "CoM6D ->  CoMXYZ2"/1, Hom/1, "CoM6D ->  CoMXYZ1"/1
  "CoM6D ->  CoMXYZ1"/1 -> MATLAB Function/1(R)
  MATLAB Function/1(rollPitchYaw) -> rollPitchYaw/1

== system torqueBalancing2015a/DesValues/State Machine StandUp/visualise inertial/Visualize hom transf4 ==
  H : Inport
  "CoM6D ->  CoMXYZ1" : Selector  NumberOfDimensions=2  InputPortWidth=7  IndexOptions=Index vector (dialog),Index vector (dialog)  Indices=[1 2 3],[1 2 3]  OutputSizes=1,1
  "CoM6D ->  CoMXYZ2" : Selector  NumberOfDimensions=2  InputPortWidth=7  IndexOptions=Index vector (dialog),Index vector (dialog)  Indices=[1 2 3],[4]  OutputSizes=1,1
  Hom : Scope
      settings: TimeRange=auto  ShowLegends=on  MaxDataPoints=5000  SaveToWorkspace=off  SaveName=ScopeData3  YMin=-0.02533  YMax=0.01393  SampleTime=-1
  MATLAB Function : MATLAB Function  TreatAsAtomicUnit=on
      settings: PermitHierarchicalResolution=ParametersOnly
  p : Scope
      settings: TimeRange=auto  MaxDataPoints=5000  SaveToWorkspace=off  SaveName=ScopeData2  YMin=-0.05005  YMax=0.09732  SampleTime=-1
  rollPitchYaw : Scope
      settings: TimeRange=auto  ShowLegends=on  MaxDataPoints=5000  SaveToWorkspace=off  YMin=-0.15453  YMax=0.04472  SampleTime=-1
  wires:
  "CoM6D ->  CoMXYZ2"/1 -> p/1
  H/1 -> "CoM6D ->  CoMXYZ2"/1, Hom/1, "CoM6D ->  CoMXYZ1"/1
  "CoM6D ->  CoMXYZ1"/1 -> MATLAB Function/1(R)
  MATLAB Function/1(rollPitchYaw) -> rollPitchYaw/1

== system torqueBalancing2015a/DesValues/State Machine StandUp/visualise inertial/Visualize hom transf5 ==
  H : Inport
  "CoM6D ->  CoMXYZ1" : Selector  NumberOfDimensions=2  InputPortWidth=7  IndexOptions=Index vector (dialog),Index vector (dialog)  Indices=[1 2 3],[1 2 3]  OutputSizes=1,1
  "CoM6D ->  CoMXYZ2" : Selector  NumberOfDimensions=2  InputPortWidth=7  IndexOptions=Index vector (dialog),Index vector (dialog)  Indices=[1 2 3],[4]  OutputSizes=1,1
  Hom : Scope
      settings: TimeRange=auto  ShowLegends=on  MaxDataPoints=5000  SaveToWorkspace=off  SaveName=ScopeData3  YMin=-0.02533  YMax=0.01393  SampleTime=-1
  MATLAB Function : MATLAB Function  TreatAsAtomicUnit=on
      settings: PermitHierarchicalResolution=ParametersOnly
  p : Scope
      settings: TimeRange=auto  MaxDataPoints=5000  SaveToWorkspace=off  SaveName=ScopeData2  YMin=-0.05005  YMax=0.09732  SampleTime=-1
  rollPitchYaw : Scope
      settings: TimeRange=auto  ShowLegends=on  MaxDataPoints=5000  SaveToWorkspace=off  YMin=-0.15453  YMax=0.04472  SampleTime=-1
  wires:
  "CoM6D ->  CoMXYZ2"/1 -> p/1
  H/1 -> "CoM6D ->  CoMXYZ2"/1, Hom/1, "CoM6D ->  CoMXYZ1"/1
  "CoM6D ->  CoMXYZ1"/1 -> MATLAB Function/1(R)
  MATLAB Function/1(rollPitchYaw) -> rollPitchYaw/1

== system torqueBalancing2015a/DesValues/State Machine StandUp/visualise inertial/Visualize hom transf6 ==
  H : Inport
  "CoM6D ->  CoMXYZ1" : Selector  NumberOfDimensions=2  InputPortWidth=7  IndexOptions=Index vector (dialog),Index vector (dialog)  Indices=[1 2 3],[1 2 3]  OutputSizes=1,1
  "CoM6D ->  CoMXYZ2" : Selector  NumberOfDimensions=2  InputPortWidth=7  IndexOptions=Index vector (dialog),Index vector (dialog)  Indices=[1 2 3],[4]  OutputSizes=1,1
  Hom : Scope
      settings: TimeRange=auto  ShowLegends=on  MaxDataPoints=5000  SaveToWorkspace=off  SaveName=ScopeData3  YMin=-0.02533  YMax=0.01393  SampleTime=-1
  MATLAB Function : MATLAB Function  TreatAsAtomicUnit=on
      settings: PermitHierarchicalResolution=ParametersOnly
  p : Scope
      settings: TimeRange=auto  MaxDataPoints=5000  SaveToWorkspace=off  SaveName=ScopeData2  YMin=-0.05005  YMax=0.09732  SampleTime=-1
  rollPitchYaw : Scope
      settings: TimeRange=auto  ShowLegends=on  MaxDataPoints=5000  SaveToWorkspace=off  YMin=-0.15453  YMax=0.04472  SampleTime=-1
  wires:
  "CoM6D ->  CoMXYZ2"/1 -> p/1
  H/1 -> "CoM6D ->  CoMXYZ2"/1, Hom/1, "CoM6D ->  CoMXYZ1"/1
  "CoM6D ->  CoMXYZ1"/1 -> MATLAB Function/1(R)
  MATLAB Function/1(rollPitchYaw) -> rollPitchYaw/1

== system torqueBalancing2015a/DesValues/State Machine StandUp/visualise inertial/Visualize hom transf7 ==
  H : Inport
  "CoM6D ->  CoMXYZ1" : Selector  NumberOfDimensions=2  InputPortWidth=7  IndexOptions=Index vector (dialog),Index vector (dialog)  Indices=[1 2 3],[1 2 3]  OutputSizes=1,1
  "CoM6D ->  CoMXYZ2" : Selector  NumberOfDimensions=2  InputPortWidth=7  IndexOptions=Index vector (dialog),Index vector (dialog)  Indices=[1 2 3],[4]  OutputSizes=1,1
  Hom : Scope
      settings: TimeRange=auto  ShowLegends=on  MaxDataPoints=5000  SaveToWorkspace=off  SaveName=ScopeData3  YMin=-0.02533  YMax=0.01393  SampleTime=-1
  MATLAB Function : MATLAB Function  TreatAsAtomicUnit=on
      settings: PermitHierarchicalResolution=ParametersOnly
  p : Scope
      settings: TimeRange=auto  MaxDataPoints=5000  SaveToWorkspace=off  SaveName=ScopeData2  YMin=-0.05005  YMax=0.09732  SampleTime=-1
  rollPitchYaw : Scope
      settings: TimeRange=auto  ShowLegends=on  MaxDataPoints=5000  SaveToWorkspace=off  YMin=-0.15453  YMax=0.04472  SampleTime=-1
  wires:
  "CoM6D ->  CoMXYZ2"/1 -> p/1
  H/1 -> "CoM6D ->  CoMXYZ2"/1, Hom/1, "CoM6D ->  CoMXYZ1"/1
  "CoM6D ->  CoMXYZ1"/1 -> MATLAB Function/1(R)
  MATLAB Function/1(rollPitchYaw) -> rollPitchYaw/1

== system torqueBalancing2015a/DesValues/State Machine StandUp/visualise inertial/Visualize hom transf8 ==
  H : Inport
  "CoM6D ->  CoMXYZ1" : Selector  NumberOfDimensions=2  InputPortWidth=7  IndexOptions=Index vector (dialog),Index vector (dialog)  Indices=[1 2 3],[1 2 3]  OutputSizes=1,1
  "CoM6D ->  CoMXYZ2" : Selector  NumberOfDimensions=2  InputPortWidth=7  IndexOptions=Index vector (dialog),Index vector (dialog)  Indices=[1 2 3],[4]  OutputSizes=1,1
  Hom : Scope
      settings: TimeRange=auto  ShowLegends=on  MaxDataPoints=5000  SaveToWorkspace=off  SaveName=ScopeData3  YMin=-0.02533  YMax=0.01393  SampleTime=-1
  MATLAB Function : MATLAB Function  TreatAsAtomicUnit=on
      settings: PermitHierarchicalResolution=ParametersOnly
  p : Scope
      settings: TimeRange=auto  MaxDataPoints=5000  SaveToWorkspace=off  SaveName=ScopeData2  YMin=-0.05005  YMax=0.09732  SampleTime=-1
  rollPitchYaw : Scope
      settings: TimeRange=auto  ShowLegends=on  MaxDataPoints=5000  SaveToWorkspace=off  YMin=-0.15453  YMax=0.04472  SampleTime=-1
  wires:
  "CoM6D ->  CoMXYZ2"/1 -> p/1
  H/1 -> "CoM6D ->  CoMXYZ2"/1, Hom/1, "CoM6D ->  CoMXYZ1"/1
  "CoM6D ->  CoMXYZ1"/1 -> MATLAB Function/1(R)
  MATLAB Function/1(rollPitchYaw) -> rollPitchYaw/1

== system torqueBalancing2015a/DesValues/State Machine StandUp/visualise inertial/l_sole_H_root_link2 ==
  qj : Inport
  Constant5 : Constant  Value=eye(4)
  Constant6 : Constant  Value=eye(4)
  Inv\* : Product  Inputs=/*  Multiplication=Matrix(*)
  Visualize hom transf4 : Subsystem
  link_name : WBToolboxLibrary/wholeBodyModel/Kinematics/Forward Kinematics  frameName=link_name  robotName=WBT_robotName  localName=WBT_modelName  wbiFile=WBT_wbiFilename  wbiList=WBT_wbiList
  root_link : WBToolboxLibrary/wholeBodyModel/Kinematics/Forward Kinematics  frameName='root_link'  robotName=WBT_robotName  localName=WBT_modelName  wbiFile=WBT_wbiFilename  wbiList=WBT_wbiList
  link_name_H_root_link : Outport
  wires:
  Constant5/1 -> link_name/1
  Inv\*/1 -> link_name_H_root_link/1  "link_name_H_root_link"
  link_name/1 -> Inv\*/1
  Constant6/1 -> root_link/1
  qj/1 -> link_name/2, root_link/2
  root_link/1 -> Visualize hom transf4/1(H), Inv\*/2

== system torqueBalancing2015a/DesValues/State Machine StandUp/visualise inertial/l_sole_H_root_link3 ==
  qj : Inport
  Constant5 : Constant  Value=eye(4)
  Constant6 : Constant  Value=eye(4)
  Inv\* : Product  Inputs=/*  Multiplication=Matrix(*)
  Visualize hom transf4 : Subsystem
  link_name : WBToolboxLibrary/wholeBodyModel/Kinematics/Forward Kinematics  frameName=link_name  robotName=WBT_robotName  localName=WBT_modelName  wbiFile=WBT_wbiFilename  wbiList=WBT_wbiList
  root_link : WBToolboxLibrary/wholeBodyModel/Kinematics/Forward Kinematics  frameName='root_link'  robotName=WBT_robotName  localName=WBT_modelName  wbiFile=WBT_wbiFilename  wbiList=WBT_wbiList
  link_name_H_root_link : Outport
  wires:
  Constant5/1 -> link_name/1
  Inv\*/1 -> link_name_H_root_link/1  "link_name_H_root_link"
  link_name/1 -> Inv\*/1
  Constant6/1 -> root_link/1
  qj/1 -> link_name/2, root_link/2
  root_link/1 -> Visualize hom transf4/1(H), Inv\*/2

== system torqueBalancing2015a/DesValues/State Machine StandUp/visualise inertial/w_H_root_link2 ==
  qj : Inport
  inertial : Inport  Port=2
  "CoM6D ->  CoMXYZ1" : Selector  NumberOfDimensions=2  InputPortWidth=7  IndexOptions=Index vector (dialog),Index vector (dialog)  Indices=[1 2 3],[1 2 3]  OutputSizes=1,1
  Constant2 : Constant  Value=eye(4)
  Constant5 : Constant  Value=eye(4)
  Constant6 : Constant  Value=eye(4)
  Inv\* : Product  Inputs=/*  Multiplication=Matrix(*)
  Inv\*1 : Product  Inputs=/*  Multiplication=Matrix(*)
  Inv\*2 : Product  Inputs=/  Multiplication=Matrix(*)
  Product : Product  Multiplication=Matrix(*)
  Selector : Selector  InputPortWidth=12  IndexOptions=Index vector (dialog)  Indices=[4 5 6 ]  OutputSizes=1
  Subsystem : Subsystem
  Switch6 : Switch  Criteria=u2 > Threshold
  USE_IMU4EST_BASE : Constant  Value=CONFIG.USE_IMU4EST_BASE
  fromImuToHomogeousTransformFCN : MATLAB Function  TreatAsAtomicUnit=on
      settings: PermitHierarchicalResolution=ParametersOnly
  holder 1 : WBToolboxLibrary/Utilities/holder 
  holder 2 : WBToolboxLibrary/Utilities/holder 
  imu : WBToolboxLibrary/wholeBodyModel/Kinematics/Forward Kinematics  frameName='imu_frame'  robotName=WBT_robotName  localName=WBT_modelName  wbiFile=WBT_wbiFilename  wbiList=WBT_wbiList
  l_sole_acc : Scope
      settings: TimeRange=60  ShowLegends=on  MaxDataPoints=5000  SaveToWorkspace=off  YMin=-4.47309  YMax=14.2668  SampleTime=-1
  link : WBToolboxLibrary/wholeBodyModel/Kinematics/Forward Kinematics  frameName=link_name  robotName=WBT_robotName  localName=WBT_modelName  wbiFile=WBT_wbiFilename  wbiList=WBT_wbiList
  root_link : WBToolboxLibrary/wholeBodyModel/Kinematics/Forward Kinematics  frameName='root_link'  robotName=WBT_robotName  localName=WBT_modelName  wbiFile=WBT_wbiFilename  wbiList=WBT_wbiList
  w_H_root : Outport
  wires:
  Constant5/1 -> imu/1
  Inv\*/1 -> holder 1/1, fromImuToHomogeousTransformFCN/1(imu_H_link), Inv\*2/1  "imu_H_link"
  imu/1 -> Inv\*/1
  Constant6/1 -> link/1
  Inv\*1/1 -> Switch6/3, fromImuToHomogeousTransformFCN/3(link_H_root)  "link_H_root"
  link/1 -> Inv\*1/1, Inv\*/2
  inertial/1 -> Selector/1, holder 2/1, fromImuToHomogeousTransformFCN/5(inertial)
  Switch6/1 -> w_H_root/1
  USE_IMU4EST_BASE/1 -> Switch6/2
  fromImuToHomogeousTransformFCN/1(w_H_root) -> Switch6/1
  Constant2/1 -> root_link/1
  qj/1 -> root_link/2, link/2, imu/2
  root_link/1 -> Inv\*1/2
  holder 1/1 -> fromImuToHomogeousTransformFCN/2(imu_H_link_0)
  holder 2/1 -> fromImuToHomogeousTransformFCN/4(inertial_0)
  Inv\*2/1 -> "CoM6D ->  CoMXYZ1"/1
  "CoM6D ->  CoMXYZ1"/1 -> Product/1  "l_sole_R_imu"
  Selector/1 -> Product/2  "imu_acce"
  Product/1 -> l_sole_acc/1
  Subsystem/1(Neck Position) -> fromImuToHomogeousTransformFCN/6(neck)
